simulink model "ONE_DOF"  (R2021b)
settings: Solver=VariableStepAuto  StartTime=0.0  StopTime=100  RelTol=1e-3
model workspace (MAT data in the model file):
  asdf = 10
  threshold = 10
libraries: aerolibanim x1, simulink x1
settings Model: SimulationMode=accelerator  Creator=darre  LastModifiedBy=darre

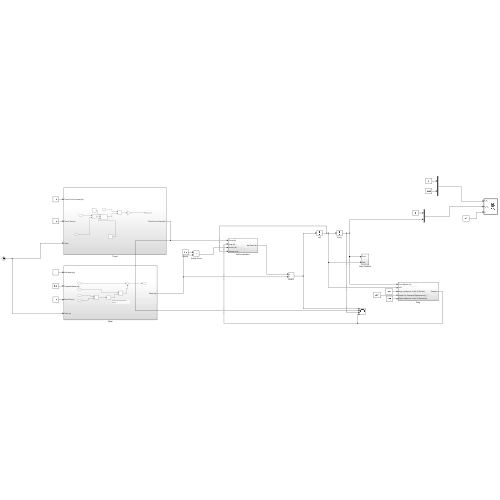
[thumbnail: Simulink's stored preview of the top-level diagram]
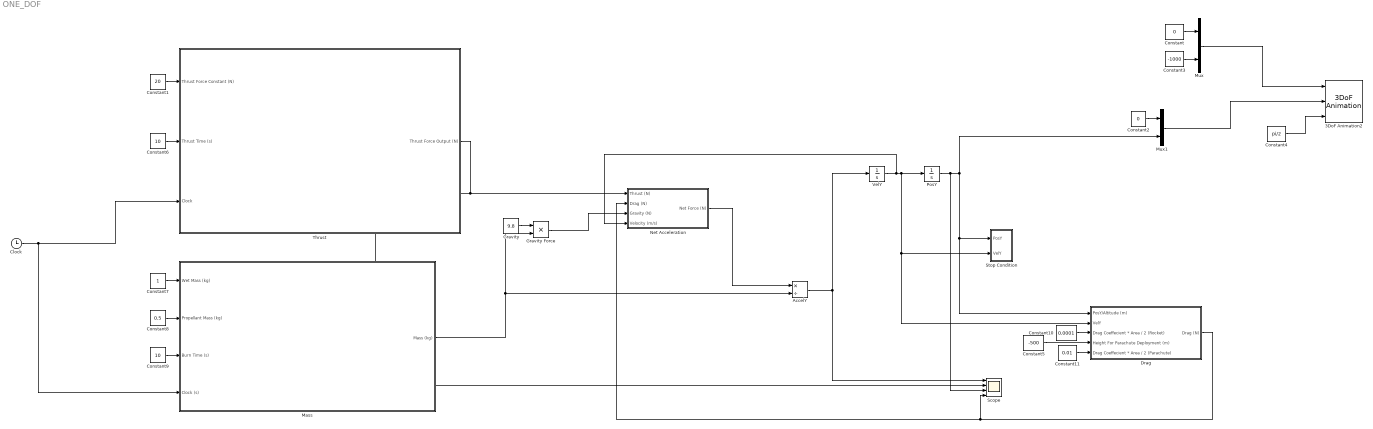
== system ONE_DOF ==
  3DoF Animation2 : aerolibanim/3DoF Animation  u1=[-1000 1000 -1000 1000 -1000 1000]  u2=0.05  u3=3  u5=Fixed position  u6=[0 1000 0]  u7=90  u8=on
      settings: SourceProductBaseCode=AE
  AccelY : Product  Inputs=*/
  Clock : Clock
  Constant : Constant  Value=0
  Constant1 : Constant  Value=20
  Constant10 : Constant  Value=0.0001
  Constant11 : Constant  Value=0.01
  Constant2 : Constant  Value=0
  Constant3 : Constant  Value=-1000
  Constant4 : Constant  Value=pi/2
  Constant5 : Constant  Value=-500
  Constant6 : Constant  Value=10
  Constant7 : Constant
  Constant8 : Constant  Value=0.5
  Constant9 : Constant  Value=10
  Drag : Subsystem
  Gravity : Constant  Value=9.8
  Gravity Force : Product
  Mass : Subsystem
  Mux : Mux  Inputs=2
  Mux1 : Mux  Inputs=2
  Net Acceleration : Subsystem
  PosY : Integrator
  Scope : Scope  NumInputPorts=4
  Stop Condition : Subsystem
  Thrust : Subsystem
  VelY : Integrator
  wires:
  Constant3/1 -> Mux/2
  Constant/1 -> Mux/1
  Mux/1 -> 3DoF Animation2/1
  Mux1/1 -> 3DoF Animation2/2
  Constant4/1 -> 3DoF Animation2/3
  PosY/1 -> Scope/3, Drag/1(PosY/Altitude (m)), Stop Condition/1(PosY), Mux1/2
  Constant2/1 -> Mux1/1
  Gravity/1 -> Gravity Force/1
  AccelY/1 -> VelY/1, Scope/1
  Constant1/1 -> Thrust/1(Thrust Force Constant (N))
  Constant6/1 -> Thrust/2(Thrust Time (s))
  Clock/1 -> Mass/4(Clock (s)), Thrust/3(Clock)
  Mass/1(Mass (kg)) -> Gravity Force/2, AccelY/2
  Constant7/1 -> Mass/1(Wet Mass (kg))
  Constant8/1 -> Mass/2(Propellant Mass (kg))
  Constant9/1 -> Mass/3(Burn Time (s))
  VelY/1 -> Net Acceleration/4(Velocity (m/s)), Drag/2(VelY), Stop Condition/2(VelY), PosY/1
  Constant10/1 -> Drag/3(Drag Coeffecient * Area / 2 (Rocket))
  Drag/1(Drag (N)) -> Scope/4, Net Acceleration/2(Drag (N))
  Thrust/1(Thrust Force Output (N)) -> Scope/2, Net Acceleration/1(Thrust (N))
  Net Acceleration/1(Net Force (N)) -> AccelY/1
  Gravity Force/1 -> Net Acceleration/3(Gravity (N))
  Constant5/1 -> Drag/4(Height For Parachute Deployment (m))
  Constant11/1 -> Drag/5(Drag Coeffecient * Area / 2 (Parachute))

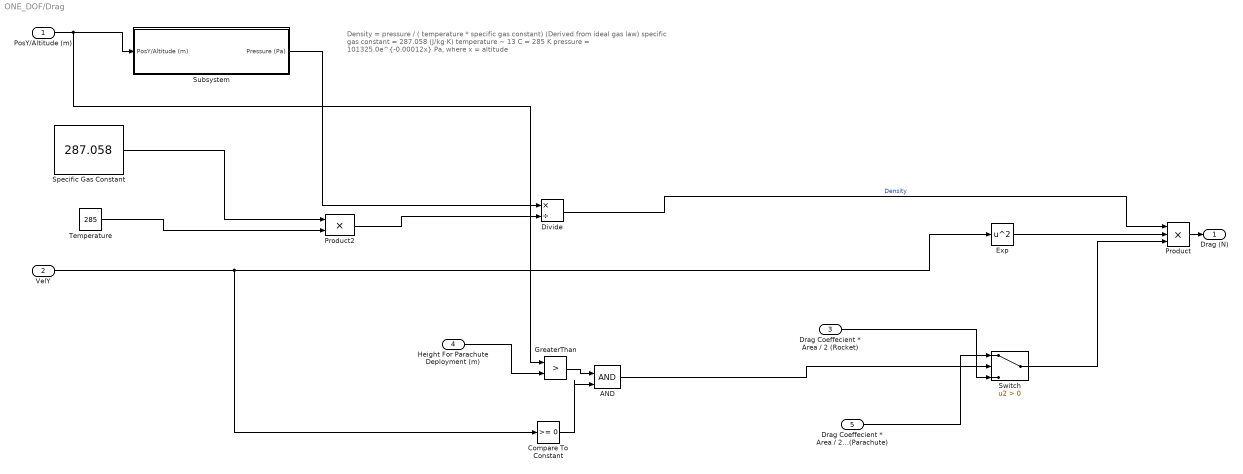
== system ONE_DOF/Drag ==
  note: Density = pressure / ( temperature * specific gas constant) (Derived from ideal gas law)
      | specific gas constant = 287.058 (J/kg·K)
      | temperature ~ 13 C = 285 K
      | pressure = 101325.0e^{-0.00012x} Pa, where x = altitude
  PosY/Altitude (m) : Inport
  VelY : Inport  Port=2
  Drag Coeffecient * Area / 2 (Rocket) : Inport  Port=3
  Height For Parachute Deployment (m) : Inport  Port=4
  Drag Coeffecient * Area / 2 (Parachute) : Inport  Port=5
  AND : Logic  IconShape=distinctive  AllPortsSameDT=off  OutDataTypeStr=boolean
  Compare To Constant : simulink/Logic and Bit Operations/Compare To Constant  relop=>=  const=0  OutDataTypeStr=boolean
  Divide : Product  Inputs=*/
  Exp : Math  Operator=square  SaturateOnIntegerOverflow=on
  GreaterThan : RelationalOperator  Operator=>  OutDataTypeStr=boolean  RndMeth=Simplest
  Product : Product  Inputs=3
  Product2 : Product
  Specific Gas Constant : Constant  Value=287.058
  Subsystem : Subsystem
  Switch : Switch  Criteria=u2 > Threshold
  Temperature : Constant  Value=285
  Drag (N) : Outport
  wires:
  Specific Gas Constant/1 -> Product2/1
  PosY/Altitude (m)/1 -> GreaterThan/1, Subsystem/1(PosY/Altitude (m))
  Subsystem/1(Pressure (Pa)) -> Divide/1
  Temperature/1 -> Product2/2
  Product2/1 -> Divide/2
  Divide/1 -> Product/1  "Density"
  Exp/1 -> Product/2
  Product/1 -> Drag (N)/1
  VelY/1 -> Compare To Constant/1, Exp/1
  Drag Coeffecient * Area / 2 (Rocket)/1 -> Switch/3
  Height For Parachute Deployment (m)/1 -> GreaterThan/2
  GreaterThan/1 -> AND/1
  Compare To Constant/1 -> AND/2
  AND/1 -> Switch/2
  Drag Coeffecient * Area / 2 (Parachute)/1 -> Switch/1
  Switch/1 -> Product/3

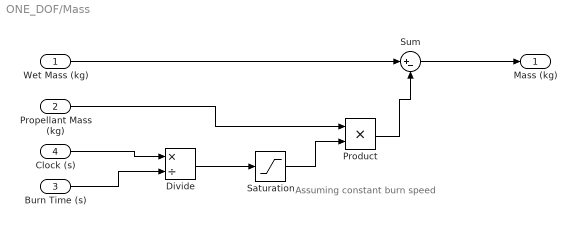
== system ONE_DOF/Mass ==
  note: Assuming constant burn speed
  Wet Mass (kg) : Inport
  Propellant Mass (kg) : Inport  Port=2
  Burn Time (s) : Inport  Port=3
  Clock (s) : Inport  Port=4
  Divide : Product  Inputs=*/
  Product : Product
  Saturation : Saturate  UpperLimit=1  LowerLimit=0
  Sum : Sum  Inputs=|+-
  Mass (kg) : Outport
  wires:
  Wet Mass (kg)/1 -> Sum/1
  Sum/1 -> Mass (kg)/1
  Propellant Mass (kg)/1 -> Product/1
  Clock (s)/1 -> Divide/1
  Divide/1 -> Saturation/1
  Product/1 -> Sum/2
  Burn Time (s)/1 -> Divide/2
  Saturation/1 -> Product/2

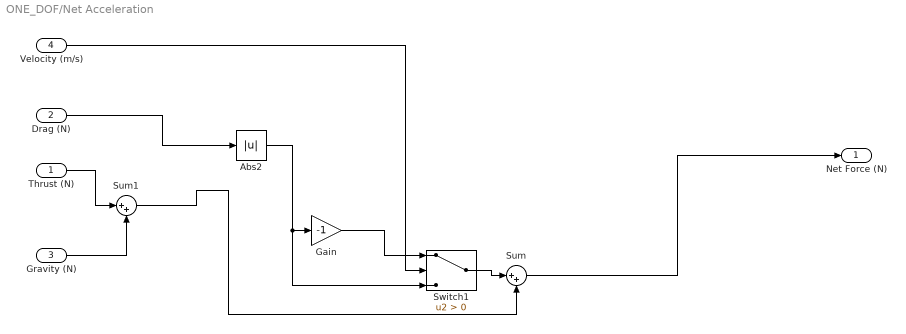
== system ONE_DOF/Net Acceleration ==
  Thrust (N) : Inport
  Drag (N) : Inport  Port=2
  Gravity (N) : Inport  Port=3
  Velocity (m/s) : Inport  Port=4
  Abs2 : Abs
  Gain : Gain  Gain=-1
  Sum : Sum  Inputs=|++
  Sum1 : Sum  Inputs=|++
  Switch1 : Switch  Criteria=u2 > Threshold
  Net Force (N) : Outport
  wires:
  Drag (N)/1 -> Abs2/1
  Thrust (N)/1 -> Sum1/1
  Abs2/1 -> Switch1/3, Gain/1
  Gain/1 -> Switch1/1
  Switch1/1 -> Sum/1
  Sum/1 -> Net Force (N)/1
  Gravity (N)/1 -> Sum1/2
  Sum1/1 -> Sum/2
  Velocity (m/s)/1 -> Switch1/2

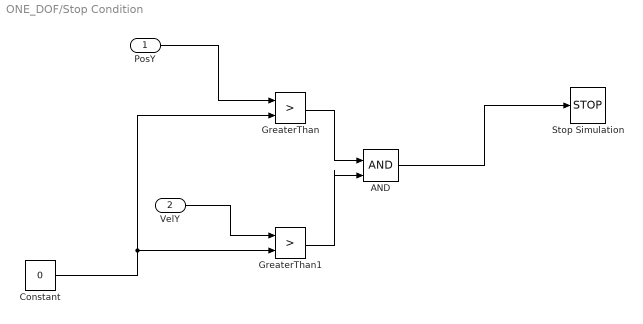
== system ONE_DOF/Stop Condition ==
  PosY : Inport
  VelY : Inport  Port=2
  AND : Logic  IconShape=distinctive  AllPortsSameDT=off  OutDataTypeStr=boolean
  Constant : Constant  Value=0
  GreaterThan : RelationalOperator  Operator=>  OutDataTypeStr=boolean  RndMeth=Simplest
  GreaterThan1 : RelationalOperator  Operator=>  OutDataTypeStr=boolean  RndMeth=Simplest
  Stop Simulation : Stop
  wires:
  GreaterThan/1 -> AND/1
  Constant/1 -> GreaterThan/2, GreaterThan1/2
  PosY/1 -> GreaterThan/1
  VelY/1 -> GreaterThan1/1
  GreaterThan1/1 -> AND/2
  AND/1 -> Stop Simulation/1

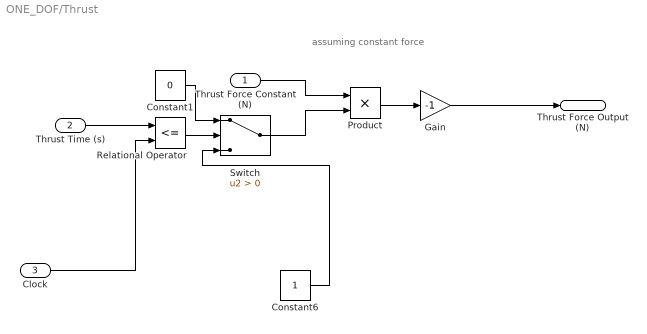
== system ONE_DOF/Thrust ==
  note: assuming constant force
  Thrust Force Constant (N) : Inport
  Thrust Time (s) : Inport  Port=2
  Clock : Inport  Port=3
  Constant1 : Constant  Value=0
  Constant6 : Constant
  Gain : Gain  Gain=-1
  Product : Product
  Relational Operator : RelationalOperator  Operator=<=  OutDataTypeStr=boolean  RndMeth=Simplest
  Switch : Switch  Criteria=u2 > Threshold
  Thrust Force Output (N) : Outport
  wires:
  Constant1/1 -> Switch/1
  Product/1 -> Gain/1
  Switch/1 -> Product/2
  Thrust Force Constant (N)/1 -> Product/1
  Relational Operator/1 -> Switch/2
  Thrust Time (s)/1 -> Relational Operator/1
  Constant6/1 -> Switch/3
  Clock/1 -> Relational Operator/2
  Gain/1 -> Thrust Force Output (N)/1

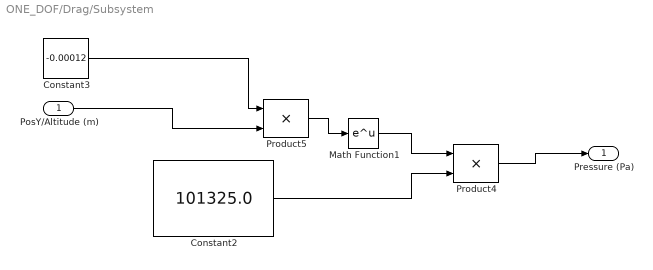
== system ONE_DOF/Drag/Subsystem ==
  PosY/Altitude (m) : Inport
  Constant2 : Constant  Value=101325.0
  Constant3 : Constant  Value=-0.00012
  Math Function1 : Math  SaturateOnIntegerOverflow=on
  Product4 : Product
  Product5 : Product
  Pressure (Pa) : Outport
  wires:
  PosY/Altitude (m)/1 -> Product5/2
  Math Function1/1 -> Product4/1
  Product4/1 -> Pressure (Pa)/1
  Constant3/1 -> Product5/1
  Product5/1 -> Math Function1/1
  Constant2/1 -> Product4/2
